simulink model "BuckConverterCascadedWithDC"  (R2021a)
settings: Solver=VariableStepAuto  StartTime=0.0  StopTime=10.0  RelTol=1e-3
undefined symbols (not defined in the file): K
libraries: simulink x2
settings Model: Creator=mithi  LastModifiedBy=Pallavi
settings DebuggingCC: UnconnectedInputMsg=none  UnconnectedOutputMsg=none  UnconnectedLineMsg=none
settings ModelReferenceCC: EnableRefExpFcnMdlSchedulingChecks=off
settings RTWCC: Description=Generic Real-Time Target  DLArmComputeVersion=20.02.1

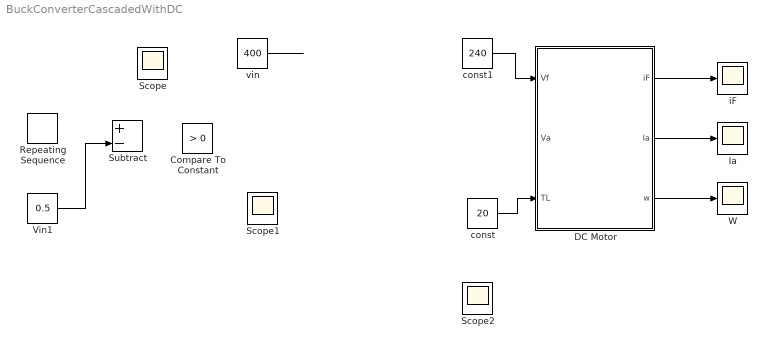
== system BuckConverterCascadedWithDC ==
  Compare To Constant : simulink/Logic and Bit Operations/Compare To Constant  relop=>  const=0  OutDataTypeStr=boolean
  DC Motor : Subsystem
  Ia : Scope
  Repeating Sequence : simulink/Sources/Repeating Sequence  rep_seq_t=[0 2]  rep_seq_y=[0 2]
  Scope : Scope
  Scope1 : Scope
  Scope2 : Scope
  Subtract : Sum  Inputs=+-
  Vin1 : Constant  Value=0.5
  W : Scope
  const : Constant  Value=20
  const1 : Constant  Value=240
  iF : Scope
  vin : Constant  Value=400
  wires:
  ? -> ?
  Vin1/1 -> Subtract/2
  vin/1 -> ?
  DC Motor/1(iF) -> iF/1
  DC Motor/2(Ia) -> Ia/1
  DC Motor/3(w) -> W/1
  const1/1 -> DC Motor/1(Vf)
  const/1 -> DC Motor/3(TL)

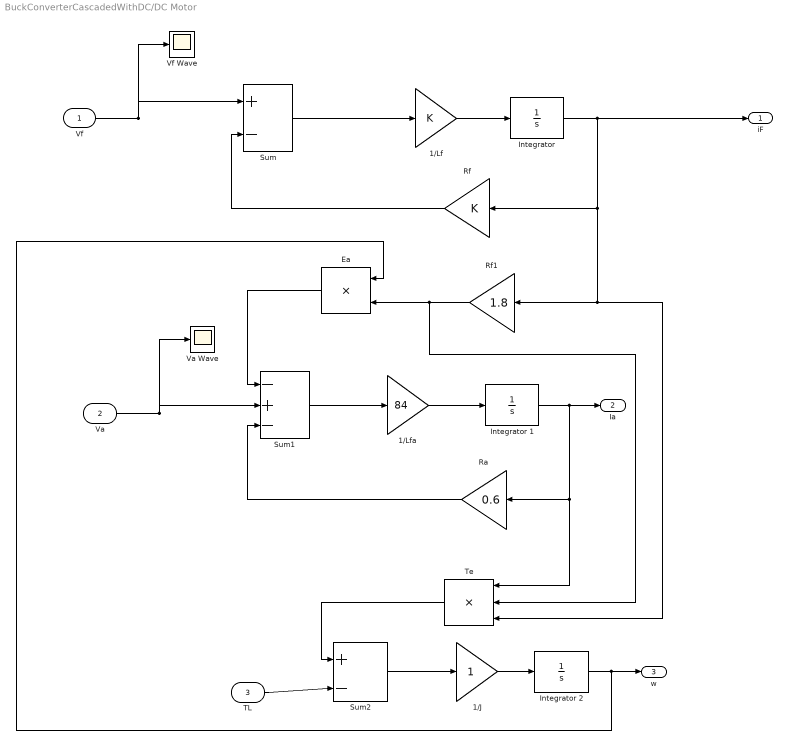
== system BuckConverterCascadedWithDC/DC Motor ==
  Vf : Inport
  Va : Inport  Port=2
  TL : Inport  Port=3
  1/J : Gain
  1/Lf : Gain  Gain=K
  1/Lfa : Gain  Gain=84
  Ea : Product
  "Integrator " : Integrator
  Integrator 1 : Integrator
  Integrator 2 : Integrator
  Ra : Gain  Gain=0.6
  Rf : Gain  Gain=K
  Rf1 : Gain  Gain=1.8
  Sum : Sum  Inputs=|+-
  Sum1 : Sum  Inputs=|-+-
  Sum2 : Sum  Inputs=|+-
  Te : Product  Inputs=3
  Va Wave : Scope
  Vf Wave : Scope
  iF : Outport
  Ia : Outport  Port=2
  w : Outport  Port=3
  wires:
  Sum2/1 -> 1/J/1
  Va/1 -> Sum1/2, Va Wave/1
  TL/1 -> Sum2/2
  Integrator 2/1 -> Ea/1, w/1
  Te/1 -> Sum2/1
  1/Lfa/1 -> Integrator 1/1
  Ea/1 -> Sum1/1
  Ra/1 -> Sum1/3
  "Integrator "/1 -> Rf1/1, Te/3, Rf/1, iF/1
  1/J/1 -> Integrator 2/1
  Rf1/1 -> Te/2, Ea/2
  Sum1/1 -> 1/Lfa/1
  1/Lf/1 -> "Integrator "/1
  Rf/1 -> Sum/2
  Integrator 1/1 -> Te/1, Ra/1, Ia/1
  Vf/1 -> Vf Wave/1, Sum/1
  Sum/1 -> 1/Lf/1
